simulink model "SWC_FDC_type"  (R2021b)
settings: Solver=FixedStepDiscrete  StartTime=0.0  StopTime=10.0  FixedStep=0.001  RelTol=1e-3
values from neighbouring files (symbols this model uses):
  DID_VCUKey = uint16(0x0202)    [vcu_local_hdr.m]
  DID_XWD = uint16(513)    [vcu_local_hdr.m]
  DIDLen_APSFunConfig = uint16(16)    [vcu_local_hdr.m]
  DIDLen_AutoLock = uint16(1)    [vcu_local_hdr.m]
  DIDLen_DKCKey = uint16(8)    [vcu_local_hdr.m]
  DIDLen_DRLDis = uint16(1)    [vcu_local_hdr.m]
  DIDLen_DynoMode = uint16(1)    [vcu_local_hdr.m]
  DIDLen_FMHTimer = uint16(1)    [vcu_local_hdr.m]
  DIDLen_LFLowPresThre = uint16(1)    [vcu_local_hdr.m]
  DIDLen_LFSensorID = uint16(4)    [vcu_local_hdr.m]
  DIDLen_LRLowPresThre = uint16(1)    [vcu_local_hdr.m]
  DIDLen_LRSensorID = uint16(4)    [vcu_local_hdr.m]
  DIDLen_RFLowPresThre = uint16(1)    [vcu_local_hdr.m]
  DIDLen_RFSensorID = uint16(4)    [vcu_local_hdr.m]
  DIDLen_RRLowPresThre = uint16(1)    [vcu_local_hdr.m]
  DIDLen_RRSensorID = uint16(4)    [vcu_local_hdr.m]
  DIDLen_SensorMode = uint16(1)    [vcu_local_hdr.m]
  DIDLen_TireSize = uint16(16)    [vcu_local_hdr.m]
  DIDLen_TPMSLearnSta = uint16(1)    [vcu_local_hdr.m]
  DIDLen_TurnLampFLThreCurr = uint16(1)    [vcu_local_hdr.m]
  DIDLen_TurnLampFRThreCurr = uint16(1)    [vcu_local_hdr.m]
  DIDLen_TurnLampRLThreCurr = uint16(1)    [vcu_local_hdr.m]
  DIDLen_TurnLampRRThreCurr = uint16(1)    [vcu_local_hdr.m]
  DIDLen_USSConfig = uint16(16)    [vcu_local_hdr.m]
  DIDLen_WhlPres = uint16(4)    [vcu_local_hdr.m]
  DIDLen_WhlSensorBattSta = uint16(1)    [vcu_local_hdr.m]
  DIDLen_WhlTmp = uint16(4)    [vcu_local_hdr.m]
  DIDLen_XWDMode = uint16(1)    [vcu_local_hdr.m]
  DIDNum_APSFunConfig = uint16(0x0903)    [vcu_local_hdr.m]
  DIDNum_AutoLock = uint16(0x0306)    [vcu_local_hdr.m]
  DIDNum_DKCKey = uint16(0x0202)    [vcu_local_hdr.m]
  DIDNum_DRLDis = uint16(0x0307)    [vcu_local_hdr.m]
  DIDNum_DynoMode = uint16(0x0203)    [vcu_local_hdr.m]
  DIDNum_FMHTimer = uint16(0x0305)    [vcu_local_hdr.m]
  DIDNum_LFLowPresThre = uint16(0x0B08)    [vcu_local_hdr.m]
  DIDNum_LFSensorID = uint16(0x0B01)    [vcu_local_hdr.m]
  DIDNum_LRLowPresThre = uint16(0x0B0A)    [vcu_local_hdr.m]
  DIDNum_LRSensorID = uint16(0x0B03)    [vcu_local_hdr.m]
  DIDNum_RFLowPresThre = uint16(0x0B09)    [vcu_local_hdr.m]
  DIDNum_RFSensorID = uint16(0x0B02)    [vcu_local_hdr.m]
  DIDNum_RRLowPresThre = uint16(0x0B0B)    [vcu_local_hdr.m]
  DIDNum_RRSensorID = uint16(0x0B04)    [vcu_local_hdr.m]
  DIDNum_SensorMode = uint16(0x0B0C)    [vcu_local_hdr.m]
  DIDNum_TireSize = uint16(0x0902)    [vcu_local_hdr.m]
  DIDNum_TPMSLearnSta = uint16(0x0B0D)    [vcu_local_hdr.m]
  DIDNum_TurnLampFLThreCurr = uint16(0x0303)    [vcu_local_hdr.m]
  DIDNum_TurnLampFRThreCurr = uint16(0x0301)    [vcu_local_hdr.m]
  DIDNum_TurnLampRLThreCurr = uint16(0x0304)    [vcu_local_hdr.m]
  DIDNum_TurnLampRRThreCurr = uint16(0x0302)    [vcu_local_hdr.m]
  DIDNum_USSConfig = uint16(0x0901)    [vcu_local_hdr.m]
  DIDNum_WhlPres = uint16(0x0B05)    [vcu_local_hdr.m]
  DIDNum_WhlSensorBattSta = uint16(0x0B07)    [vcu_local_hdr.m]
  DIDNum_WhlTmp = uint16(0x0B06)    [vcu_local_hdr.m]
  DIDNum_XWDMode = uint16(0x0201)    [vcu_local_hdr.m]
  DIDVCUKeyLength = uint16(8)    [vcu_local_hdr.m]
  ENUM_DRIVETRAIN_AWD = uint8(  2  )    [vcu_local_hdr.m]
  ENUM_DRIVETRAIN_FWD = uint8(  1  )    [vcu_local_hdr.m]
  ENUM_DRIVETRAIN_RWD = uint8(  0  )    [vcu_local_hdr.m]
  ENUM_REGENLEVEL_INVALID = uint8(  7  )    [vcu_local_hdr.m]
  ENUM_REGENLEVEL_LV1 = uint8(  1  )    [vcu_local_hdr.m]
  ENUM_REGENLEVEL_LV2 = uint8(  2  )    [vcu_local_hdr.m]
  ENUM_REGENLEVEL_LV3 = uint8(  3  )    [vcu_local_hdr.m]
  ENUM_REGENLEVEL_LV4 = uint8(  4  )    [vcu_local_hdr.m]
  ENUM_REGENLEVEL_LV5 = uint8(  5  )    [vcu_local_hdr.m]
  ENUM_REGENLEVEL_OFF = uint8(  0  )    [vcu_local_hdr.m]
  ENUM_REGENLEVEL_OPD = uint8(  6  )    [vcu_local_hdr.m]
  ENUM_TPMSLearnStatus_LEARNED = uint8(  1  )    [vcu_local_hdr.m]
  ENUM_TPMSLearnStatus_LEARNFAIL = uint8(  2  )    [vcu_local_hdr.m]
  ENUM_TPMSLearnStatus_NOTLEARN = uint8(  0  )    [vcu_local_hdr.m]
  ENUM_TPMSSTA_FAT = uint8(  8  )    [vcu_local_hdr.m]
  ENUM_TPMSSTA_LOWBATTERY = uint8(  2  )    [vcu_local_hdr.m]
  FALSE = boolean( 0 )    [vcu_local_hdr.m]
  ONE_INT = uint8(1)    [vcu_local_hdr.m]
  P_boolean = 0.0    [APPTypes.sldd]
  TRUE = boolean( 1 )    [vcu_local_hdr.m]
  ZERO_FLOAT = single(0)    [vcu_local_hdr.m]
  ZERO_INT = uint8(0)    [vcu_local_hdr.m]
undefined symbols (not defined in the file or in its folder): f32_ApsOutVehSpdSig, KHAL_DKCDecryptEnable_flg_ovrdflg, KHAL_DKCDecryptEnable_flg_ovrdval, KHAL_RandomNumberY1_enum, KHAL_RandomNumberY2_enum, KHAL_RandomNumberY_ovrdflg, KHAL_THCMAPTCWarningDTC_flg_ovrdflg, KHAL_THCMAPTCWarningDTC_flg_ovrdval, KHAL_TPMSRESBUTT_flg_ovrdflg, KHAL_TPMSRESBUTT_flg_ovrdval, R_DIDWriteCDD_CSOP_DIDSet_APSFunConfig, R_DIDWriteCDD_CSOP_DIDSet_AutoLock, R_DIDWriteCDD_CSOP_DIDSet_DKCKey, R_DIDWriteCDD_CSOP_DIDSet_DRLDis, R_DIDWriteCDD_CSOP_DIDSet_DynoMode, R_DIDWriteCDD_CSOP_DIDSet_FMHTimer, R_DIDWriteCDD_CSOP_DIDSet_LFLowPresThre, R_DIDWriteCDD_CSOP_DIDSet_LFSensorID, R_DIDWriteCDD_CSOP_DIDSet_LRLowPresThre, R_DIDWriteCDD_CSOP_DIDSet_LRSensorID, R_DIDWriteCDD_CSOP_DIDSet_RFLowPresThre, R_DIDWriteCDD_CSOP_DIDSet_RFSensorID, R_DIDWriteCDD_CSOP_DIDSet_RRLowPresThre, R_DIDWriteCDD_CSOP_DIDSet_RRSensorID, R_DIDWriteCDD_CSOP_DIDSet_SensorMode, R_DIDWriteCDD_CSOP_DIDSet_TireSize, R_DIDWriteCDD_CSOP_DIDSet_TPMSLearnSta, R_DIDWriteCDD_CSOP_DIDSet_TurnLampFLThreCurr, R_DIDWriteCDD_CSOP_DIDSet_TurnLampFRThreCurr, R_DIDWriteCDD_CSOP_DIDSet_TurnLampRLThreCurr, R_DIDWriteCDD_CSOP_DIDSet_TurnLampRRThreCurr, R_DIDWriteCDD_CSOP_DIDSet_USSConfig, R_DIDWriteCDD_CSOP_DIDSet_WhlPres, R_DIDWriteCDD_CSOP_DIDSet_WhlSensorBattSta, R_DIDWriteCDD_CSOP_DIDSet_WhlTmp, R_DIDWriteCDD_CSOP_DIDSet_XWDMode, R_E2E_CAN3_VCU1_CSOP_Write_CAN3_VCU1, R_E2E_CAN3_VCU1_toNIDEC_CSOP_Write_CAN3_VCU1_toNIDEC, R_E2E_CAN4_VCU1_CSOP_Write_CAN4_VCU1, R_FDCCDD_Inner_CSOP_FDC_AppCallSleep, R_HALINCDD_CSOP_PAS_Handler, R_HALINCDD_CSOP_UDS_Main, R_HALOUT_APS_CSOP_ApsOutput, R_HALOUTCDD_CSOP_AppNmStateReq, R_HALOUTCDD_CSOP_SetAcoreRebootCmdACK, R_HALOUTCDD_CSOP_SetSysPwrStat, R_HALOUTCDD_CSOP_SleepRequest, R_IOExpOUT_CDD_CSOP_IOExpSetVal, R_NVMReadCDD_Inner_NVM_ReadOperation, R_NVMWriteCDD_Inner_NVM_WriteOperation, R_UDSCDD_CSOP_DdmRestartOperationCycle, R_WDGCDD_CSOP_Call_Watchdog, R_WDGCDD_CSOP_Call_WDG_AppEnd, R_WDGCDD_CSOP_Call_WDG_AppStart, u16_DIDLen_APSFunConfig, u16_DIDLen_AutoLock, u16_DIDLen_DKCKey, u16_DIDLen_DRLDis, u16_DIDLen_DynoMode, u16_DIDLen_FMHTimer ... (+83)
libraries: simulink x215, FVT_lib x139, hcu_lib x21, hdlsllib x9, app x1, halin x1, halout x1, inp x1, outp x1
(part 12 of 12)

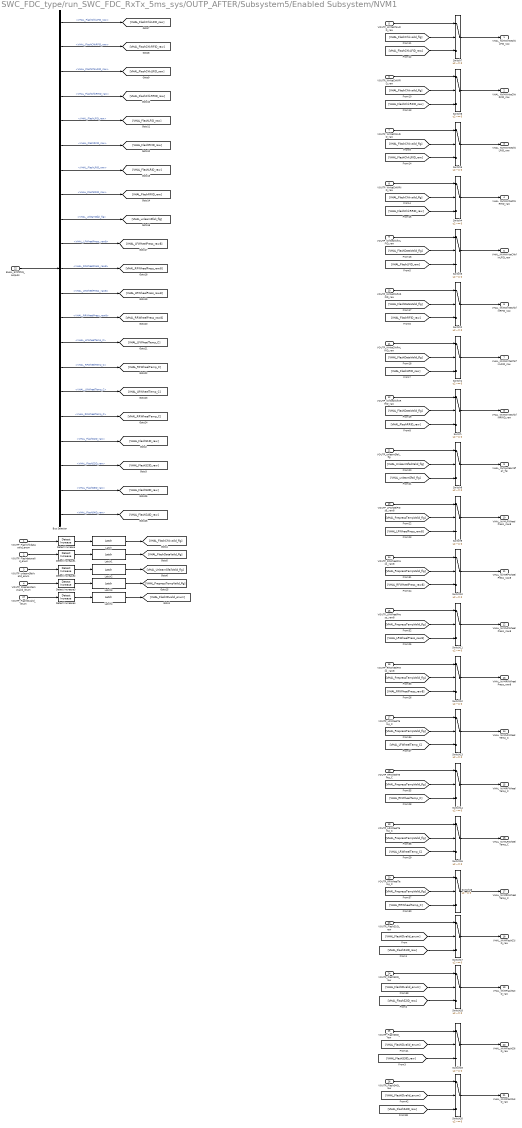
== system SWC_FDC_type/run_SWC_FDC_RxTx_5ms_sys/OUTP_AFTER/Subsystem5/Enabled Subsystem/NVM1 ==
  VOUTP_Flashchkdatavalid_enum : Inport
  VOUTP_Flashdatavalid_enum : Inport  Port=2
  VOUTP_unlearnSfailvalid_enum : Inport  Port=3
  VOUTP_Prepresstempvalid_enum : Inport  Port=4
  VOUTP_WriteChkLFID_raw : Inport  Port=5
  VOUTP_WriteChkRFID_raw : Inport  Port=6
  VOUTP_WriteChkLRID_raw : Inport  Port=7
  VOUTP_WriteChkRRID_raw : Inport  Port=8
  VOUTP_WriteChkfinLFID_raw : Inport  Port=9
  VOUTP_WriteChkfinRFID_raw : Inport  Port=10
  VOUTP_WriteChkfinLRID_raw : Inport  Port=11
  VOUTP_WriteChkfinRRID_raw : Inport  Port=12
  VOUTP_LFWheelPress_raw8 : Inport  Port=13
  VOUTP_RFWheelPress_raw8 : Inport  Port=14
  VOUTP_LRWheelPress_raw8 : Inport  Port=15
  VOUTP_RRWheelPress_raw8 : Inport  Port=16
  VOUTP_LFWheelTemp_C : Inport  Port=17
  VOUTP_RFWheelTemp_C : Inport  Port=18
  VOUTP_LRWheelTemp_C : Inport  Port=19
  VOUTP_RRWheelTemp_C : Inport  Port=20
  VOUTP_unlearnSfali_flg : Inport  Port=21
  BHAL_SYSTPMS_outputs : Inport  Port=22
  VOUTP_FlashS1ID_raw : Inport  Port=23
  VOUTP_FlashS2ID_raw : Inport  Port=24
  VOUTP_FlashS3ID_raw : Inport  Port=25
  VOUTP_FlashS4ID_raw : Inport  Port=26
  VOUTP_FlashIDvalid_enum : Inport  Port=27
  Bus Selector : BusSelector  OutputSignals=VHAL_FlashChkLFID_raw,VHAL_FlashChkRFID_raw,VHAL_FlashChkLRID_raw,VHAL_FlashChkRRID_raw,VHAL_FlashLFID_raw,VHAL_FlashRFID_raw,VHAL_FlashLRID_raw,VHAL_FlashRRID_raw,VHAL_unlearnSfali_flg,VHAL_LFWheelPress_raw8,VHAL_RFWheelPress_raw8,VHAL_LRWheelPress_raw8,VHAL_RRWheelPress_raw8,VHAL_LFWheelTemp_C,VHAL_RFWheelTemp_C,VHAL_LRWheelTemp_C,VHAL_RRWheelTemp_C,VHAL_FlashS1ID_raw,VHAL_FlashS2ID_raw,VHAL_FlashS3ID_raw,VHAL_FlashS4ID_raw
  Detect Increase{,1..4} (5 alike) : simulink/Logic and Bit Operations/Detect Increase  vinit=0.0  OutDataTypeStr=boolean
  Latch{,1..4} (5 alike) : hcu_lib/Basic_Blocks/Latch
  Switch{,1..20} (21 alike) : Switch  Criteria=u2 ~= 0
  VHAL_NVMWriteChkLFID_raw : Outport
  VHAL_NVMWriteChkRFID_raw : Outport  Port=2
  VHAL_NVMWriteChkLRID_raw : Outport  Port=3
  VHAL_NVMWriteChkRRID_raw : Outport  Port=4
  VHAL_NVMWriteChkfinLFID_raw : Outport  Port=5
  VHAL_NVMWriteChkfinRFID_raw : Outport  Port=6
  VHAL_NVMWriteChkfinLRID_raw : Outport  Port=7
  VHAL_NVMWriteChkfinRRID_raw : Outport  Port=8
  VHAL_NVMunlearnSfali_flg : Outport  Port=9
  VHAL_NVMLFWheelPress_raw8 : Outport  Port=10
  VHAL_NVMRFWheelPress_raw8 : Outport  Port=11
  VHAL_NVMLRWheelPress_raw8 : Outport  Port=12
  VHAL_NVMRRWheelPress_raw8 : Outport  Port=13
  VHAL_NVMLFWheelTemp_C : Outport  Port=14
  VHAL_NVMRFWheelTemp_C : Outport  Port=15
  VHAL_NVMLRWheelTemp_C : Outport  Port=16
  VHAL_NVMRRWheelTemp_C : Outport  Port=17
  VHAL_NVMFlashS1ID_raw : Outport  Port=18
  VHAL_NVMFlashS2ID_raw : Outport  Port=19
  VHAL_NVMFlashS3ID_raw : Outport  Port=20
  VHAL_NVMFlashS4ID_raw : Outport  Port=21
  wires:
  Bus Selector/2 -> [VHAL_FlashChkRFID_raw]  "<VHAL_FlashChkRFID_raw>"
  Bus Selector/1 -> [VHAL_FlashChkLFID_raw]  "<VHAL_FlashChkLFID_raw>"
  Bus Selector/11 -> [VHAL_RFWheelPress_raw8]  "<VHAL_RFWheelPress_raw8>"
  Bus Selector/3 -> [VHAL_FlashChkLRID_raw]  "<VHAL_FlashChkLRID_raw>"
  Bus Selector/7 -> [VHAL_FlashLRID_raw]  "<VHAL_FlashLRID_raw>"
  Bus Selector/5 -> [VHAL_FlashLFID_raw]  "<VHAL_FlashLFID_raw>"
  Bus Selector/6 -> [VHAL_FlashRFID_raw]  "<VHAL_FlashRFID_raw>"
  Bus Selector/8 -> [VHAL_FlashRRID_raw]  "<VHAL_FlashRRID_raw>"
  Bus Selector/14 -> [VHAL_LFWheelTemp_C]  "<VHAL_LFWheelTemp_C>"
  Bus Selector/9 -> [VHAL_unlearnSfali_flg]  "<VHAL_unlearnSfali_flg>"
  Bus Selector/13 -> [VHAL_RRWheelPress_raw8]  "<VHAL_RRWheelPress_raw8>"
  Bus Selector/4 -> [VHAL_FlashChkRRID_raw]  "<VHAL_FlashChkRRID_raw>"
  Bus Selector/12 -> [VHAL_LRWheelPress_raw8]  "<VHAL_LRWheelPress_raw8>"
  BHAL_SYSTPMS_outputs/1 -> Bus Selector/1
  Bus Selector/15 -> [VHAL_RFWheelTemp_C]  "<VHAL_RFWheelTemp_C>"
  Bus Selector/10 -> [VHAL_LFWheelPress_raw8]  "<VHAL_LFWheelPress_raw8>"
  Bus Selector/17 -> [VHAL_RRWheelTemp_C]  "<VHAL_RRWheelTemp_C>"
  Bus Selector/16 -> [VHAL_LRWheelTemp_C]  "<VHAL_LRWheelTemp_C>"
  Switch/1 -> VHAL_NVMWriteChkfinRRID_raw/1
  Switch1/1 -> VHAL_NVMWriteChkfinLRID_raw/1
  Switch2/1 -> VHAL_NVMWriteChkfinRFID_raw/1
  Switch3/1 -> VHAL_NVMWriteChkfinLFID_raw/1
  Switch4/1 -> VHAL_NVMWriteChkRRID_raw/1
  Switch5/1 -> VHAL_NVMWriteChkLRID_raw/1
  Switch6/1 -> VHAL_NVMWriteChkRFID_raw/1
  Switch7/1 -> VHAL_NVMWriteChkLFID_raw/1
  Switch8/1 -> VHAL_NVMunlearnSfali_flg/1
  VOUTP_WriteChkRFID_raw/1 -> Switch6/1
  VOUTP_WriteChkLFID_raw/1 -> Switch7/1
  VOUTP_WriteChkfinLFID_raw/1 -> Switch3/1
  VOUTP_WriteChkRRID_raw/1 -> Switch4/1
  VOUTP_WriteChkLRID_raw/1 -> Switch5/1
  VOUTP_WriteChkfinRRID_raw/1 -> Switch/1
  VOUTP_WriteChkfinLRID_raw/1 -> Switch1/1
  [VHAL_FlashRRID_raw] -> Switch/3
  VOUTP_WriteChkfinRFID_raw/1 -> Switch2/1
  [VHAL_FlashChkvalid_flg] -> Switch7/2
  [VHAL_FlashChkvalid_flg] -> Switch4/2
  [VHAL_FlashRFID_raw] -> Switch2/3
  [VHAL_FlashLFID_raw] -> Switch3/3
  [VHAL_FlashChkLFID_raw] -> Switch7/3
  [VHAL_FlashChkLRID_raw] -> Switch5/3
  [VHAL_FlashDataValid_flg] -> Switch1/2
  [VHAL_FlashChkRRID_raw] -> Switch4/3
  [VHAL_FlashDataValid_flg] -> Switch/2
  [VHAL_FlashDataValid_flg] -> Switch3/2
  [VHAL_FlashChkvalid_flg] -> Switch5/2
  [VHAL_FlashDataValid_flg] -> Switch2/2
  [VHAL_FlashChkRFID_raw] -> Switch6/3
  [VHAL_FlashLRID_raw] -> Switch1/3
  [VHAL_FlashChkvalid_flg] -> Switch6/2
  VOUTP_Prepresstempvalid_enum/1 -> Detect Increase3/1
  VOUTP_unlearnSfailvalid_enum/1 -> Detect Increase2/1
  VOUTP_Flashdatavalid_enum/1 -> Detect Increase1/1
  VOUTP_Flashchkdatavalid_enum/1 -> Detect Increase/1
  Latch3/1 -> [VHAL_PrepressTempValid_flg]
  Detect Increase/1 -> Latch/1
  Detect Increase2/1 -> Latch2/1
  Latch1/1 -> [VHAL_FlashDataValid_flg]
  Latch2/1 -> [VHAL_UnlearnSfailValid_flg]
  Latch/1 -> [VHAL_FlashChkvalid_flg]
  Detect Increase3/1 -> Latch3/1
  Detect Increase1/1 -> Latch1/1
  [VHAL_unlearnSfali_flg] -> Switch8/3
  VOUTP_unlearnSfali_flg/1 -> Switch8/1
  [VHAL_UnlearnSfailValid_flg] -> Switch8/2
  VOUTP_RRWheelTemp_C/1 -> Switch16/1
  VOUTP_LFWheelTemp_C/1 -> Switch13/1
  VOUTP_RFWheelTemp_C/1 -> Switch14/1
  VOUTP_LRWheelTemp_C/1 -> Switch15/1
  VOUTP_LFWheelPress_raw8/1 -> Switch9/1
  Switch16/1 -> VHAL_NVMRRWheelTemp_C/1
  Switch13/1 -> VHAL_NVMLFWheelTemp_C/1
  [VHAL_LRWheelTemp_C] -> Switch15/3
  Switch15/1 -> VHAL_NVMLRWheelTemp_C/1
  Switch14/1 -> VHAL_NVMRFWheelTemp_C/1
  [VHAL_PrepressTempValid_flg] -> Switch16/2
  VOUTP_RFWheelPress_raw8/1 -> Switch10/1
  Switch9/1 -> VHAL_NVMLFWheelPress_raw8/1
  Switch10/1 -> VHAL_NVMRFWheelPress_raw8/1
  [VHAL_LFWheelTemp_C] -> Switch13/3
  Switch11/1 -> VHAL_NVMLRWheelPress_raw8/1
  [VHAL_PrepressTempValid_flg] -> Switch9/2
  [VHAL_RFWheelTemp_C] -> Switch14/3
  [VHAL_RRWheelPress_raw8] -> Switch12/3
  Switch12/1 -> VHAL_NVMRRWheelPress_raw8/1
  [VHAL_PrepressTempValid_flg] -> Switch12/2
  [VHAL_PrepressTempValid_flg] -> Switch14/2
  [VHAL_LFWheelPress_raw8] -> Switch9/3
  [VHAL_LRWheelPress_raw8] -> Switch11/3
  [VHAL_RFWheelPress_raw8] -> Switch10/3
  [VHAL_PrepressTempValid_flg] -> Switch15/2
  VOUTP_LRWheelPress_raw8/1 -> Switch11/1
  [VHAL_PrepressTempValid_flg] -> Switch10/2
  [VHAL_RRWheelTemp_C] -> Switch16/3
  [VHAL_PrepressTempValid_flg] -> Switch13/2
  [VHAL_PrepressTempValid_flg] -> Switch11/2
  VOUTP_RRWheelPress_raw8/1 -> Switch12/1
  Detect Increase4/1 -> Latch4/1
  Latch4/1 -> [VHAL_FlashIDvalid_enum]
  VOUTP_FlashIDvalid_enum/1 -> Detect Increase4/1
  [VHAL_FlashS1ID_raw] -> Switch17/3
  [VHAL_FlashIDvalid_enum] -> Switch17/2
  Switch17/1 -> VHAL_NVMFlashS1ID_raw/1
  VOUTP_FlashS1ID_raw/1 -> Switch17/1
  Bus Selector/18 -> [VHAL_FlashS1ID_raw]  "<VHAL_FlashS1ID_raw>"
  Bus Selector/19 -> [VHAL_FlashS2ID_raw]  "<VHAL_FlashS2ID_raw>"
  Bus Selector/20 -> [VHAL_FlashS3ID_raw]  "<VHAL_FlashS3ID_raw>"
  Bus Selector/21 -> [VHAL_FlashS4ID_raw]  "<VHAL_FlashS4ID_raw>"
  [VHAL_FlashS2ID_raw] -> Switch18/3
  Switch18/1 -> VHAL_NVMFlashS2ID_raw/1
  VOUTP_FlashS2ID_raw/1 -> Switch18/1
  [VHAL_FlashIDvalid_enum] -> Switch18/2
  Switch19/1 -> VHAL_NVMFlashS3ID_raw/1
  [VHAL_FlashS3ID_raw] -> Switch19/3
  [VHAL_FlashIDvalid_enum] -> Switch19/2
  VOUTP_FlashS3ID_raw/1 -> Switch19/1
  Switch20/1 -> VHAL_NVMFlashS4ID_raw/1
  [VHAL_FlashS4ID_raw] -> Switch20/3
  [VHAL_FlashIDvalid_enum] -> Switch20/2
  VOUTP_FlashS4ID_raw/1 -> Switch20/1

== system SWC_FDC_type/run_SWC_FDC_RxTx_5ms_sys/OUTP_AFTER/Subsystem5/Enabled Subsystem/Subsystem ==
  VOUTP_DiagFMHT_s : Inport
  Add1 : Sum  Inputs=+-
  Constant45 : Constant  Value=10
  Gain4 : Gain  Gain=1/5
  Saturation : Saturate  UpperLimit=150  LowerLimit=5
  Out1 : Outport
  wires:
  VOUTP_DiagFMHT_s/1 -> Add1/1
  Constant45/1 -> Add1/2
  Gain4/1 -> Out1/1
  Saturation/1 -> Gain4/1
  Add1/1 -> Saturation/1

== system SWC_FDC_type/run_SWC_FDC_RxTx_5ms_sys/Subsystem2/DKC2/DKC Decryption and Unpack/DKCReVehData ==
  Byte_4 : Inport
  BitwiseAND : simulink/Logic and Bit Operations/Bitwise Operator  logicop=AND  UseBitMask=off  NumInputPorts=2  BitMask=bin2dec('11011001')  BitMaskRealWorld=Stored Integer
  BitwiseOR : simulink/Logic and Bit Operations/Bitwise Operator  logicop=OR  UseBitMask=off  BitMask=bin2dec('11011001')  BitMaskRealWorld=Stored Integer
  Constant : Constant  Value=(2^4-1)
  LeftShift : ArithShift  BitShiftDirection=Left
  RightShift : ArithShift  BitShiftNumber=4  BitShiftDirection=Right
  UnitConverter : DataTypeConversion  OutDataTypeStr=uint8
  UnitConverter1 : DataTypeConversion  OutDataTypeStr=uint8
  VHAL_DKCReVehData_enum : Outport
  wires:
  BitwiseOR/1 -> RightShift/1
  RightShift/1 -> BitwiseAND/1
  UnitConverter/1 -> BitwiseAND/2
  Constant/1 -> UnitConverter/1
  BitwiseAND/1 -> VHAL_DKCReVehData_enum/1
  LeftShift/1 -> BitwiseOR/1
  UnitConverter1/1 -> LeftShift/1
  Byte_4/1 -> UnitConverter1/1

== system SWC_FDC_type/run_SWC_FDC_RxTx_5ms_sys/Subsystem2/DKC2/DKC Decryption and Unpack/DKCRemotePW ==
  Byte_3 : Inport
  BitwiseAND : simulink/Logic and Bit Operations/Bitwise Operator  logicop=AND  UseBitMask=off  NumInputPorts=2  BitMask=bin2dec('11011001')  BitMaskRealWorld=Stored Integer
  BitwiseOR : simulink/Logic and Bit Operations/Bitwise Operator  logicop=OR  UseBitMask=off  BitMask=bin2dec('11011001')  BitMaskRealWorld=Stored Integer
  Constant : Constant  Value=(2^5-1)
  LeftShift : ArithShift  BitShiftDirection=Left
  RightShift : ArithShift  BitShiftDirection=Right
  UnitConverter : DataTypeConversion  OutDataTypeStr=uint8
  UnitConverter1 : DataTypeConversion  OutDataTypeStr=uint8
  VHAL_DKCRemotePW_enum : Outport
  wires:
  BitwiseOR/1 -> RightShift/1
  RightShift/1 -> BitwiseAND/1
  UnitConverter/1 -> BitwiseAND/2
  Constant/1 -> UnitConverter/1
  BitwiseAND/1 -> VHAL_DKCRemotePW_enum/1
  LeftShift/1 -> BitwiseOR/1
  UnitConverter1/1 -> LeftShift/1
  Byte_3/1 -> UnitConverter1/1

== system SWC_FDC_type/run_SWC_FDC_RxTx_5ms_sys/Subsystem2/DKC2/DKC Decryption and Unpack/PCommandToBCM ==
  Byte_0 : Inport
  BitwiseAND : simulink/Logic and Bit Operations/Bitwise Operator  logicop=AND  UseBitMask=off  NumInputPorts=2  BitMask=bin2dec('11011001')  BitMaskRealWorld=Stored Integer
  BitwiseOR : simulink/Logic and Bit Operations/Bitwise Operator  logicop=OR  UseBitMask=off  BitMask=bin2dec('11011001')  BitMaskRealWorld=Stored Integer
  Constant : Constant  Value=(2^4-1)
  LeftShift : ArithShift  BitShiftDirection=Left
  RightShift : ArithShift  BitShiftNumber=4  BitShiftDirection=Right
  UnitConverter : DataTypeConversion  OutDataTypeStr=uint8
  UnitConverter1 : DataTypeConversion  OutDataTypeStr=uint8
  VHAL_PCommandToBCM_enum : Outport
  wires:
  BitwiseOR/1 -> RightShift/1
  RightShift/1 -> BitwiseAND/1
  UnitConverter/1 -> BitwiseAND/2
  Constant/1 -> UnitConverter/1
  BitwiseAND/1 -> VHAL_PCommandToBCM_enum/1
  LeftShift/1 -> BitwiseOR/1
  UnitConverter1/1 -> LeftShift/1
  Byte_0/1 -> UnitConverter1/1

== system SWC_FDC_type/run_SWC_FDC_RxTx_5ms_sys/Subsystem2/DKC2/DKC Decryption and Unpack/PCommandToPTG ==
  Byte_1 : Inport
  BitwiseAND : simulink/Logic and Bit Operations/Bitwise Operator  logicop=AND  UseBitMask=off  NumInputPorts=2  BitMask=bin2dec('11011001')  BitMaskRealWorld=Stored Integer
  BitwiseOR : simulink/Logic and Bit Operations/Bitwise Operator  logicop=OR  UseBitMask=off  BitMask=bin2dec('11011001')  BitMaskRealWorld=Stored Integer
  Constant : Constant  Value=(2^3-1)
  LeftShift : ArithShift  BitShiftDirection=Left
  RightShift : ArithShift  BitShiftDirection=Right
  UnitConverter : DataTypeConversion  OutDataTypeStr=uint8
  UnitConverter1 : DataTypeConversion  OutDataTypeStr=uint8
  VHAL_PCommandToPTG_enum : Outport
  wires:
  BitwiseOR/1 -> RightShift/1
  RightShift/1 -> BitwiseAND/1
  UnitConverter/1 -> BitwiseAND/2
  Constant/1 -> UnitConverter/1
  BitwiseAND/1 -> VHAL_PCommandToPTG_enum/1
  LeftShift/1 -> BitwiseOR/1
  UnitConverter1/1 -> LeftShift/1
  Byte_1/1 -> UnitConverter1/1

== system SWC_FDC_type/run_SWC_FDC_RxTx_5ms_sys/Subsystem2/DKC2/DKC Decryption and Unpack/PDKeyAreaLockUnlock ==
  Byte_1 : Inport
  BitwiseAND : simulink/Logic and Bit Operations/Bitwise Operator  logicop=AND  UseBitMask=off  NumInputPorts=2  BitMask=bin2dec('11011001')  BitMaskRealWorld=Stored Integer
  BitwiseOR : simulink/Logic and Bit Operations/Bitwise Operator  logicop=OR  UseBitMask=off  BitMask=bin2dec('11011001')  BitMaskRealWorld=Stored Integer
  Constant : Constant  Value=(2^2-1)
  LeftShift : ArithShift  BitShiftDirection=Left
  RightShift : ArithShift  BitShiftNumber=6  BitShiftDirection=Right
  UnitConverter : DataTypeConversion  OutDataTypeStr=uint8
  UnitConverter1 : DataTypeConversion  OutDataTypeStr=uint8
  VHAL_PDKeyAreaLockUnlock_enum : Outport
  wires:
  BitwiseOR/1 -> RightShift/1
  RightShift/1 -> BitwiseAND/1
  UnitConverter/1 -> BitwiseAND/2
  Constant/1 -> UnitConverter/1
  BitwiseAND/1 -> VHAL_PDKeyAreaLockUnlock_enum/1
  LeftShift/1 -> BitwiseOR/1
  UnitConverter1/1 -> LeftShift/1
  Byte_1/1 -> UnitConverter1/1

== system SWC_FDC_type/run_SWC_FDC_RxTx_5ms_sys/Subsystem2/DKC2/DKC Decryption and Unpack/PDKeyAreaPS ==
  Byte_1 : Inport
  BitwiseAND : simulink/Logic and Bit Operations/Bitwise Operator  logicop=AND  UseBitMask=off  NumInputPorts=2  BitMask=bin2dec('11011001')  BitMaskRealWorld=Stored Integer
  BitwiseOR : simulink/Logic and Bit Operations/Bitwise Operator  logicop=OR  UseBitMask=off  BitMask=bin2dec('11011001')  BitMaskRealWorld=Stored Integer
  Constant : Constant  Value=(2^2-1)
  LeftShift : ArithShift  BitShiftDirection=Left
  RightShift : ArithShift  BitShiftNumber=4  BitShiftDirection=Right
  UnitConverter : DataTypeConversion  OutDataTypeStr=uint8
  UnitConverter1 : DataTypeConversion  OutDataTypeStr=uint8
  VHAL_PDKeyAreaPS_enum : Outport
  wires:
  BitwiseOR/1 -> RightShift/1
  RightShift/1 -> BitwiseAND/1
  UnitConverter/1 -> BitwiseAND/2
  Constant/1 -> UnitConverter/1
  BitwiseAND/1 -> VHAL_PDKeyAreaPS_enum/1
  LeftShift/1 -> BitwiseOR/1
  UnitConverter1/1 -> LeftShift/1
  Byte_1/1 -> UnitConverter1/1

== system SWC_FDC_type/run_SWC_FDC_RxTx_5ms_sys/Subsystem2/DKC2/DKC Decryption and Unpack/PDKeyAreaPTG ==
  Byte_3 : Inport
  BitwiseAND : simulink/Logic and Bit Operations/Bitwise Operator  logicop=AND  UseBitMask=off  NumInputPorts=2  BitMask=bin2dec('11011001')  BitMaskRealWorld=Stored Integer
  BitwiseOR : simulink/Logic and Bit Operations/Bitwise Operator  logicop=OR  UseBitMask=off  BitMask=bin2dec('11011001')  BitMaskRealWorld=Stored Integer
  Constant : Constant  Value=(2^2-1)
  LeftShift : ArithShift  BitShiftDirection=Left
  RightShift : ArithShift  BitShiftNumber=6  BitShiftDirection=Right
  UnitConverter : DataTypeConversion  OutDataTypeStr=uint8
  UnitConverter1 : DataTypeConversion  OutDataTypeStr=uint8
  VHAL_PDKeyAreaPTG_enum : Outport
  wires:
  BitwiseOR/1 -> RightShift/1
  RightShift/1 -> BitwiseAND/1
  UnitConverter/1 -> BitwiseAND/2
  Constant/1 -> UnitConverter/1
  BitwiseAND/1 -> VHAL_PDKeyAreaPTG_enum/1
  LeftShift/1 -> BitwiseOR/1
  UnitConverter1/1 -> LeftShift/1
  Byte_3/1 -> UnitConverter1/1

== system SWC_FDC_type/run_SWC_FDC_RxTx_5ms_sys/Subsystem2/DKC2/DKC Decryption and Unpack/PDKeyWelcome ==
  Byte_0 : Inport
  BitwiseAND : simulink/Logic and Bit Operations/Bitwise Operator  logicop=AND  UseBitMask=off  NumInputPorts=2  BitMask=bin2dec('11011001')  BitMaskRealWorld=Stored Integer
  BitwiseOR : simulink/Logic and Bit Operations/Bitwise Operator  logicop=OR  UseBitMask=off  BitMask=bin2dec('11011001')  BitMaskRealWorld=Stored Integer
  Constant : Constant  Value=(2^4-1)
  LeftShift : ArithShift  BitShiftDirection=Left
  RightShift : ArithShift  BitShiftDirection=Right
  UnitConverter : DataTypeConversion  OutDataTypeStr=uint8
  UnitConverter1 : DataTypeConversion  OutDataTypeStr=uint8
  VHAL_PDKeyWelcome_enum : Outport
  wires:
  BitwiseOR/1 -> RightShift/1
  RightShift/1 -> BitwiseAND/1
  UnitConverter/1 -> BitwiseAND/2
  Constant/1 -> UnitConverter/1
  BitwiseAND/1 -> VHAL_PDKeyWelcome_enum/1
  LeftShift/1 -> BitwiseOR/1
  UnitConverter1/1 -> LeftShift/1
  Byte_0/1 -> UnitConverter1/1

== system SWC_FDC_type/run_SWC_FDC_RxTx_5ms_sys/Subsystem2/DKC2/DKC Decryption and Unpack/PDkeyShowIVI ==
  Byte_2 : Inport
  BitwiseAND : simulink/Logic and Bit Operations/Bitwise Operator  logicop=AND  UseBitMask=off  NumInputPorts=2  BitMask=bin2dec('11011001')  BitMaskRealWorld=Stored Integer
  BitwiseOR : simulink/Logic and Bit Operations/Bitwise Operator  logicop=OR  UseBitMask=off  BitMask=bin2dec('11011001')  BitMaskRealWorld=Stored Integer
  Constant : Constant  Value=(2^4-1)
  LeftShift : ArithShift  BitShiftDirection=Left
  RightShift : ArithShift  BitShiftNumber=4  BitShiftDirection=Right
  UnitConverter : DataTypeConversion  OutDataTypeStr=uint8
  UnitConverter1 : DataTypeConversion  OutDataTypeStr=uint8
  VHAL_PDkeyShowIVI_enum : Outport
  wires:
  BitwiseOR/1 -> RightShift/1
  RightShift/1 -> BitwiseAND/1
  UnitConverter/1 -> BitwiseAND/2
  Constant/1 -> UnitConverter/1
  BitwiseAND/1 -> VHAL_PDkeyShowIVI_enum/1
  LeftShift/1 -> BitwiseOR/1
  UnitConverter1/1 -> LeftShift/1
  Byte_2/1 -> UnitConverter1/1

== system SWC_FDC_type/run_SWC_FDC_RxTx_5ms_sys/Subsystem2/DKC2/DKC Decryption and Unpack/PKeyMiss ==
  Byte_3 : Inport
  BitwiseAND : simulink/Logic and Bit Operations/Bitwise Operator  logicop=AND  UseBitMask=off  NumInputPorts=2  BitMask=bin2dec('11011001')  BitMaskRealWorld=Stored Integer
  BitwiseOR : simulink/Logic and Bit Operations/Bitwise Operator  logicop=OR  UseBitMask=off  BitMask=bin2dec('11011001')  BitMaskRealWorld=Stored Integer
  Constant : Constant  Value=(2^1-1)
  LeftShift : ArithShift  BitShiftDirection=Left
  RightShift : ArithShift  BitShiftNumber=5  BitShiftDirection=Right
  UnitConverter : DataTypeConversion  OutDataTypeStr=uint8
  UnitConverter1 : DataTypeConversion  OutDataTypeStr=uint8
  VHAL_PKeyMiss_flg : Outport
  wires:
  BitwiseOR/1 -> RightShift/1
  RightShift/1 -> BitwiseAND/1
  UnitConverter/1 -> BitwiseAND/2
  Constant/1 -> UnitConverter/1
  BitwiseAND/1 -> VHAL_PKeyMiss_flg/1
  LeftShift/1 -> BitwiseOR/1
  UnitConverter1/1 -> LeftShift/1
  Byte_3/1 -> UnitConverter1/1

== system SWC_FDC_type/run_SWC_FDC_RxTx_5ms_sys/Subsystem2/DKC2/DKC Decryption and Unpack/PKeyMode ==
  Byte_2 : Inport
  BitwiseAND : simulink/Logic and Bit Operations/Bitwise Operator  logicop=AND  UseBitMask=off  NumInputPorts=2  BitMask=bin2dec('11011001')  BitMaskRealWorld=Stored Integer
  BitwiseOR : simulink/Logic and Bit Operations/Bitwise Operator  logicop=OR  UseBitMask=off  BitMask=bin2dec('11011001')  BitMaskRealWorld=Stored Integer
  Constant : Constant  Value=(2^4-1)
  LeftShift : ArithShift  BitShiftDirection=Left
  RightShift : ArithShift  BitShiftDirection=Right
  UnitConverter : DataTypeConversion  OutDataTypeStr=uint8
  UnitConverter1 : DataTypeConversion  OutDataTypeStr=uint8
  VHAL_PKeyMode_enum : Outport
  wires:
  BitwiseOR/1 -> RightShift/1
  RightShift/1 -> BitwiseAND/1
  UnitConverter/1 -> BitwiseAND/2
  Constant/1 -> UnitConverter/1
  BitwiseAND/1 -> VHAL_PKeyMode_enum/1
  LeftShift/1 -> BitwiseOR/1
  UnitConverter1/1 -> LeftShift/1
  Byte_2/1 -> UnitConverter1/1

== system SWC_FDC_type/run_SWC_FDC_RxTx_5ms_sys/Subsystem2/DKC2/DKC Decryption and Unpack/PUIDLowPower ==
  Byte_1 : Inport
  BitwiseAND : simulink/Logic and Bit Operations/Bitwise Operator  logicop=AND  UseBitMask=off  NumInputPorts=2  BitMask=bin2dec('11011001')  BitMaskRealWorld=Stored Integer
  BitwiseOR : simulink/Logic and Bit Operations/Bitwise Operator  logicop=OR  UseBitMask=off  BitMask=bin2dec('11011001')  BitMaskRealWorld=Stored Integer
  Constant : Constant  Value=(2^1-1)
  LeftShift : ArithShift  BitShiftDirection=Left
  RightShift : ArithShift  BitShiftNumber=3  BitShiftDirection=Right
  UnitConverter : DataTypeConversion  OutDataTypeStr=uint8
  UnitConverter1 : DataTypeConversion  OutDataTypeStr=uint8
  VHAL_PUIDLowPower_flg : Outport
  wires:
  BitwiseOR/1 -> RightShift/1
  RightShift/1 -> BitwiseAND/1
  UnitConverter/1 -> BitwiseAND/2
  Constant/1 -> UnitConverter/1
  BitwiseAND/1 -> VHAL_PUIDLowPower_flg/1
  LeftShift/1 -> BitwiseOR/1
  UnitConverter1/1 -> LeftShift/1
  Byte_1/1 -> UnitConverter1/1

== matlab function SWC_FDC_type/run_SWC_FDC_RxTx_5ms_sys/Halin_CDD/Halin_TPMS/Subsystem/CRC8_Caculation/MATLAB Function ==
  data: msg_raw input; CRC_Out output
function CRC_Out= fcn(msg_raw)

message = uint16(0);
remainder = uint16(0);
divisor = 0b1000001110000000u16;
divisorDegree = 8;
messageLength = 8;
CRC_raw = uint16(0);
%if divisor polynomial should be an input, use this:
%divisor = bitshift(divisor,divisorDegree-1);

for i = 1:8

    message = bitshift(msg_raw(i),divisorDegree);
    remainder = bitxor(CRC_raw,message);

    for k = 1:messageLength
        if bitget(remainder,messageLength+divisorDegree)
            remainder = bitxor(remainder,divisor);
        end
        remainder = bitshift(remainder,1);
    end
    CRC_raw = remainder;

end

CRC_Out = bitshift(CRC_raw,-divisorDegree);

== stateflow chart SWC_FDC_type/run_SWC_FDC_RxTx_5ms_sys/Halin_CDD/TPM_Scheduler ==
  state Task_10ms
    (default) -> (junction 8) : {
        | counter = 0;
        | }
    Task_10ms -> (junction 8) : {
        | counter++;
        | }
    (junction 8) -> (junction 5) [order 1] : [counter%%2 == 0]  /* 10ms trigger #1*/
    (junction 8) -> (junction 6) [order 2]
    (junction 5) -> (junction 7) : {
        | trig_TPM_10ms1;
        | }
    (junction 7) -> (junction 6)
  data: counter local double
  events: trig_TPM_10ms1 output FUNCTION_CALL_EVENT

== stateflow chart SWC_FDC_type/run_SWC_FDC_RxTx_5ms_sys/hcu_main_sched ==
  state Main_Scheduler
    (default) -> (junction 31) : {
        |   Sys_Init_done = FALSE;
        |   trig_Read_NVM_00;
        |   trig_ReadIMUOffset_00;
        | }
    Main_Scheduler -> (junction 31) : {Sys_Init_done = TRUE;}
    (junction 31) -> (junction 34) [order 1] : [
        |    Sys_Init_done &&...
        |    !VHAL_FusionSchedReq_flg
        | ]
    (junction 31) -> (junction 38) [order 2]
    (junction 34) -> (junction 36) : {
        |     trig_WDG;
        |     trig_GetNMID;
        |     trig_GetDID;
        |     trig_HAL_IN_10;
        |     trig_HAL_CDD_10_1;
        |     trig_HAL_DKC_10_2;
        |     trig_HAL_DKC_10_3;
        |     trig_INP_20;
        |     trig_APP_30;
        |     trig_OUTP_40;
        |     trig_OUTP_AFTER_40_1;
        |     trig_HAL_OUT_50;
        |     trig_HAL_OUTAFTER_50_1;
        |    }
    (junction 36) -> (junction 38)
  (default) -> Main_Scheduler
  data: VHAL_FusionSchedReq_flg input; Sys_Init_done local double; FALSE parameter; TRUE parameter
  events: trig_Read_NVM_00 output FUNCTION_CALL_EVENT; trig_ReadIMUOffset_00 output FUNCTION_CALL_EVENT; trig_WDG output FUNCTION_CALL_EVENT; trig_GetNMID output FUNCTION_CALL_EVENT; trig_GetDID output FUNCTION_CALL_EVENT; trig_HAL_IN_10 output FUNCTION_CALL_EVENT; trig_HAL_CDD_10_1 output FUNCTION_CALL_EVENT; trig_HAL_DKC_10_2 output FUNCTION_CALL_EVENT; trig_HAL_DKC_10_3 output FUNCTION_CALL_EVENT; trig_INP_20 output FUNCTION_CALL_EVENT; trig_APP_30 output FUNCTION_CALL_EVENT; trig_OUTP_40 output FUNCTION_CALL_EVENT; trig_OUTP_AFTER_40_1 output FUNCTION_CALL_EVENT; trig_HAL_OUT_50 output FUNCTION_CALL_EVENT; trig_HAL_OUTAFTER_50_1 output FUNCTION_CALL_EVENT
